simulink model "flightControlSystem"  (R2021a)
settings: Solver=ode3  StartTime=0  StopTime=TFinal  FixedStep=Ts  RelTol=1e-3  EnableMultiTasking=on
undefined symbols (not defined in the file): BINARIZATION_THRESHOLD, CHANGE_DERIVATIVE_ERROR_THRESHOLD_CURVE, CHANGE_DERIVATIVE_ERROR_THRESHOLD_STRAIGHT, codertarget, COG_X, COG_Y, Controller, DELAY_LANDING, DERIVATIVE_GAIN, DILATE_KERNEL, DiscIntNeverNeededParam, Discrete, DISK_KERNEL, Estimator, FLAG_WAIT_FOR_HOVERING, FOV_CURVE, FOV_STRAIGHT, FRAME_SIZE_HEIGHT, FRAME_SIZE_WIDTH, g, G_B_GAIN, GAIN_LANDING, GAIN_TRACK, init, MAX_RADIUS_CROWN_CURVE, MAX_RADIUS_CROWN_STRAIGHT, MIN_RADIUS_CROWN_CURVE, MIN_RADIUS_CROWN_STRAIGHT, Sensors, strel, Time, TIME_HOLD, Ts, var_acc_angle_N, var_bias_gyr_N, var_gyro_p_N, Vehicle, Z_HIGH, Z_LOW
libraries: simulink x39, ctrlSharedLib x4, sharedtransform x3, visionmorphops x2, parrotlib x1
(part 2 of 3)

== system flightControlSystem/Control System/State Estimator/XY Position Estimator ==
  opticalFlow_datin : Inport
  controlModePosVSOrient_flagin : Inport  Port=2
  sensorIMU_datin : Inport  Port=3
  Z_estimin : Inport  Port=4
  dz_estimin : Inport  Port=5
  orient_estimin : Inport  Port=6
  Angular velocity : Inport  Port=7
  EstimatorVelocity : Subsystem
  EstimatorXYPosition : Subsystem
  XY_estimout : Outport  VectorParamsAs1DForOutWhenUnconnected=off
  dxy_estimout : Outport  Port=2  VectorParamsAs1DForOutWhenUnconnected=off
  wires:
  EstimatorXYPosition/1(XY_estimout) -> XY_estimout/1
  dz_estimin/1 -> EstimatorXYPosition/4(dz_estimin)
  controlModePosVSOrient_flagin/1 -> EstimatorXYPosition/3(controlModePosVSOrient_flagin)
  Z_estimin/1 -> EstimatorVelocity/2(Z_estimin)
  sensorIMU_datin/1 -> EstimatorVelocity/3(sensorIMU_datin)
  opticalFlow_datin/1 -> EstimatorVelocity/1(opticalFlow_datin)
  EstimatorVelocity/1(dxy_estimout) -> dxy_estimout/1, EstimatorXYPosition/1(dxy_estimin)
  orient_estimin/1 -> EstimatorXYPosition/2(orient_estimin), EstimatorVelocity/4(orient_estimin)
  Angular velocity/1 -> EstimatorVelocity/5(angular velocity)

== system flightControlSystem/Control System/Path Planning/Non linear Path Planner/X_PLANNER ==
  x_estimated : Inport
  error_x : Inport  Port=2
  flag_end_marker : Inport  Port=3
  flag_end_marker_to_controller : Inport  Port=4
  flag_track : Inport  Port=5
  flag_hover : Inport  Port=6
  change_threshold : Inport  Port=7
  Cast To Double1 : DataTypeConversion  OutDataTypeStr=double
  Chart1 : Stateflow chart  TreatAsAtomicUnit=on
  "x_derivative_contribute " : Subsystem
  x_linear_contribute : Stateflow chart  TreatAsAtomicUnit=on
  x_planned : Outport  VectorParamsAs1DForOutWhenUnconnected=off
  wires:
  "x_derivative_contribute "/1(derivative_x_part) -> Chart1/1(dev_part)
  x_estimated/1 -> Cast To Double1/1
  flag_end_marker_to_controller/1 -> Chart1/3(flag_end_marker_to_controller)
  error_x/1 -> "x_derivative_contribute "/1(error_x), x_linear_contribute/1(error)
  Cast To Double1/1 -> Chart1/4(x_estimated)
  flag_track/1 -> Chart1/5(flag_track), x_linear_contribute/3(flag_track)
  x_linear_contribute/1(linear_part) -> Chart1/2(lin_part)
  flag_end_marker/1 -> Chart1/6(flag_end_marker), x_linear_contribute/2(flag_end_marker)
  Chart1/1(x_planned) -> x_planned/1
  flag_hover/1 -> Chart1/7(flag_hover)
  change_threshold/1 -> "x_derivative_contribute "/2(change_threshold)

== system flightControlSystem/Control System/Path Planning/Non linear Path Planner/Y_PLANNER ==
  flag_track : Inport
  flag_end_marker_to_controller : Inport  Port=2
  flag_end_marker : Inport  Port=3
  error_y : Inport  Port=4
  y_estimated : Inport  Port=5
  flag_hover : Inport  Port=6
  change_threshold : Inport  Port=7
  Cast To Double1 : DataTypeConversion  OutDataTypeStr=double
  Chart1 : Stateflow chart  TreatAsAtomicUnit=on
  "y_derivative_contribute " : Subsystem
  y_linear_contribute : Stateflow chart  TreatAsAtomicUnit=on
  y_planned : Outport  VectorParamsAs1DForOutWhenUnconnected=off
  wires:
  error_y/1 -> y_linear_contribute/1(error), "y_derivative_contribute "/2(error_y)
  "y_derivative_contribute "/1(derivative_y_part) -> Chart1/1(dev_part)
  y_estimated/1 -> Cast To Double1/1
  flag_end_marker/1 -> Chart1/5(flag_end_marker), y_linear_contribute/2(flag_end_marker)
  flag_track/1 -> Chart1/4(flag_track), y_linear_contribute/3(flag_track)
  y_linear_contribute/1(linear_part) -> Chart1/2(lin_part)
  Cast To Double1/1 -> Chart1/6(y_estimated)
  flag_end_marker_to_controller/1 -> Chart1/3(flag_end_marker_to_controller)
  Chart1/1(y_planned) -> y_planned/1
  flag_hover/1 -> Chart1/7(flag_hover)
  change_threshold/1 -> "y_derivative_contribute "/1(change_threshold)

== system flightControlSystem/Control System/Path Planning/Non linear Path Planner/Z PLANNER ==
  error_x : Inport
  flag_end_marker : Inport  Port=2
  error_y : Inport  Port=3
  flag_hover : Inport  Port=4
  Chart : Stateflow chart  TreatAsAtomicUnit=on
  Delay1 : Delay  DelayLength=DELAY_LANDING
  Display : Display
  MATLAB Function : MATLAB Function  TreatAsAtomicUnit=on
  z_planned : Outport  VectorParamsAs1DForOutWhenUnconnected=off
  flag_end_marker_to_controller : Outport  Port=2  VectorParamsAs1DForOutWhenUnconnected=off
  wires:
  error_y/1 -> MATLAB Function/2(error_y)
  error_x/1 -> MATLAB Function/1(error_x)
  flag_end_marker/1 -> Chart/2(flag_end_marker), MATLAB Function/3(flag_end_marker)
  MATLAB Function/2(norm_error) -> Delay1/1
  Delay1/1 -> MATLAB Function/4(norm_error_prev)
  MATLAB Function/1(norm_error_tot) -> Display/1, Chart/1(norm_error)
  Chart/1(z_planned) -> z_planned/1
  Chart/2(flag_end_marker_to_controller) -> flag_end_marker_to_controller/1
  flag_hover/1 -> Chart/3(flag_hover)

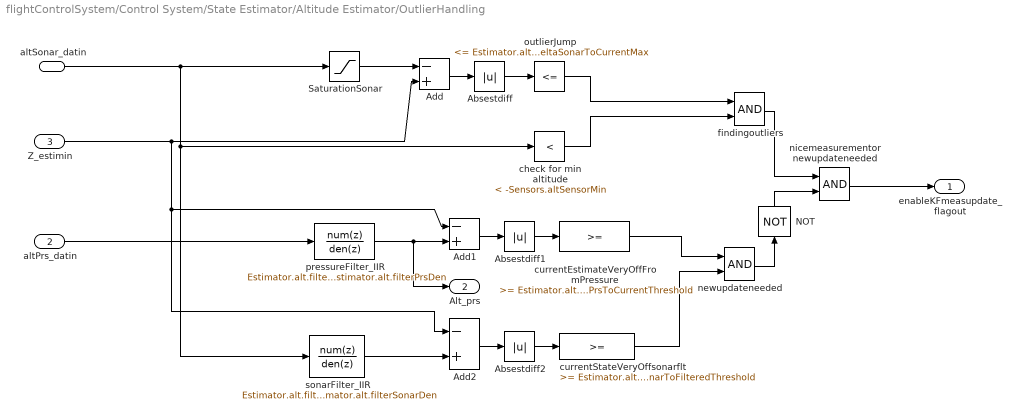
== system flightControlSystem/Control System/State Estimator/Altitude Estimator/OutlierHandling ==
  altSonar_datin : Inport
  altPrs_datin : Inport  Port=2
  Z_estimin : Inport  Port=3
  Absestdiff : Abs
  Absestdiff1 : Abs
  Absestdiff2 : Abs
  Add : Sum  Inputs=-+
  Add1 : Sum  Inputs=-+
  Add2 : Sum  Inputs=-+
  NOT : Logic  Operator=NOT  IconShape=distinctive  AllPortsSameDT=off  OutDataTypeStr=boolean
  SaturationSonar : Saturate  UpperLimit=-Sensors.altSensorMin  LowerLimit=-inf
  check for min altitude : simulink/Logic and Bit Operations/Compare To Constant  relop=<  const=-Sensors.altSensorMin  OutDataTypeStr=boolean
  currentEstimateVeryOffFromPressure : simulink/Logic and Bit Operations/Compare To Constant  relop=>=  const=Estimator.alt.deltaPrsToCurrentThreshold  OutDataTypeStr=boolean
  currentStateVeryOffsonarflt : simulink/Logic and Bit Operations/Compare To Constant  relop=>=  const=Estimator.alt.deltaSonarToFilteredThreshold  OutDataTypeStr=boolean
  findingoutliers : Logic  AllPortsSameDT=off  OutDataTypeStr=boolean
  newupdateneeded : Logic  AllPortsSameDT=off  OutDataTypeStr=boolean
  nicemeasurementor newupdateneeded : Logic  AllPortsSameDT=off  OutDataTypeStr=boolean
  outlierJump : simulink/Logic and Bit Operations/Compare To Constant  relop=<=  const=Estimator.alt.deltaSonarToCurrentMax  OutDataTypeStr=boolean
  pressureFilter_IIR : DiscreteFilter  Numerator=Estimator.alt.filterPrsNum  Denominator=Estimator.alt.filterPrsDen
  sonarFilter_IIR : DiscreteFilter  Numerator=Estimator.alt.filterSonarNum  Denominator=Estimator.alt.filterSonarDen
  enableKFmeasupdate_flagout : Outport  VectorParamsAs1DForOutWhenUnconnected=off
  Alt_prs : Outport  Port=2  VectorParamsAs1DForOutWhenUnconnected=off
  wires:
  Add1/1 -> Absestdiff1/1
  nicemeasurementor newupdateneeded/1 -> enableKFmeasupdate_flagout/1
  findingoutliers/1 -> nicemeasurementor newupdateneeded/1
  check for min altitude/1 -> findingoutliers/2
  outlierJump/1 -> findingoutliers/1
  SaturationSonar/1 -> Add/1
  Absestdiff/1 -> outlierJump/1
  Add/1 -> Absestdiff/1
  newupdateneeded/1 -> NOT/1
  Absestdiff2/1 -> currentStateVeryOffsonarflt/1
  altSonar_datin/1 -> SaturationSonar/1, sonarFilter_IIR/1, check for min altitude/1
  currentEstimateVeryOffFromPressure/1 -> newupdateneeded/1
  Z_estimin/1 -> Add1/1, Add2/1, Add/2
  Add2/1 -> Absestdiff2/1
  currentStateVeryOffsonarflt/1 -> newupdateneeded/2
  pressureFilter_IIR/1 -> Alt_prs/1, Add1/2
  altPrs_datin/1 -> pressureFilter_IIR/1
  sonarFilter_IIR/1 -> Add2/2
  Absestdiff1/1 -> currentEstimateVeryOffFromPressure/1
  NOT/1 -> nicemeasurementor newupdateneeded/2

== system flightControlSystem/Control System/State Estimator/Attitude Estimator/Pitch_Kalman ==
  note: Gyroscope's bias is susceptible to factors like "temperature" and "Gyro bias stability" and it
      | can vary during the flight. It is therefore estimated using this Kalman filter making use of Accelerometer data
  note: Linear Kalman filter is used for the Pitch and Roll estimation.
      | The states are the corresponding Euler angle and Angular rate bias respectively
  axyz : Inport
  pitch_rate : Inport  Port=2
  enable_update : Inport  Port=3
  Demux : Demux  Outputs=2
  Gain2 : Gain  Gain=1/g
  Kalman Filter : ctrlSharedLib/Kalman Filter  TimeDomain=Discrete-Time  UseCurrentEstimator=on  ModelSource=Individual A, B, C, D matrices  ModelSourceVariable=ss(0.95,1,1,0,1)  A=[1 -Ts;0 1]  B=[Ts;0]  C=[1 0]  D=0  NumberOfStates=1  NumberOfInputs=1  NumberOfOutputs=1  InitialEstimateSource=Dialog  X0=0  P0=10  UseK=off  UseGH=off  NumberOfProcessNoiseInputs=1  G=1  TimeInvariantG=on  H=0  TimeInvariantH=on  Q=[var_gyro_p_N,0;0,var_bias_gyr_N]  TimeInvariantQ=on  R=var_acc_angle_N  TimeInvariantR=on  N=0  TimeInvariantN=on  AddInputPort=on  AddEnablePort=on  OutputEstimatedY=off  OutputP=off  Ts=Ts
  Selector1 : Selector  InputPortWidth=3  IndexOptions=Index vector (dialog)  Indices=[1]  OutputSizes=1
  Trigonometric Function1 : Trigonometry  Operator=asin
  single : DataTypeConversion  OutDataTypeStr=single
  single1 : DataTypeConversion  OutDataTypeStr=single
  pitch : Outport
  gyro_y_bias : Outport  Port=2
  wires:
  Kalman Filter/1 -> Demux/1
  Demux/1 -> single1/1
  Gain2/1 -> Trigonometric Function1/1
  Trigonometric Function1/1 -> Kalman Filter/2
  Selector1/1 -> Gain2/1
  axyz/1 -> Selector1/1
  pitch_rate/1 -> Kalman Filter/1
  enable_update/1 -> Kalman Filter/3
  Demux/2 -> single/1
  single/1 -> gyro_y_bias/1
  single1/1 -> pitch/1

== system flightControlSystem/Control System/State Estimator/Attitude Estimator/Roll_Kalman ==
  note: Linear Kalman filter is used for the Pitch and Roll estimation.
      | The states are the corresponding Euler angle and Angular rate bias respectively
  note: Gyroscope's bias is susceptible to factors like "temperature" and "Gyro bias stability" and it
      | can vary during the flight. It is therefore estimated using the Kalman filter making use of accelerometer data
  axyz : Inport
  roll_rate : Inport  Port=2
  enable_update : Inport  Port=3
  Data Type Conversion : DataTypeConversion
  Data Type Conversion1 : DataTypeConversion
  Demux : Demux  Outputs=3
  Demux1 : Demux  Outputs=2
  Divide : Product  Inputs=*/
  Kalman Filter : ctrlSharedLib/Kalman Filter  TimeDomain=Discrete-Time  UseCurrentEstimator=on  ModelSource=Individual A, B, C, D matrices  ModelSourceVariable=ss(0.95,1,1,0,1)  A=[1 -Ts;0 1]  B=[Ts;0]  C=[1 0]  D=0  NumberOfStates=1  NumberOfInputs=1  NumberOfOutputs=1  InitialEstimateSource=Dialog  X0=0  P0=10  UseK=off  UseGH=off  NumberOfProcessNoiseInputs=1  G=1  TimeInvariantG=on  H=0  TimeInvariantH=on  Q=[var_gyro_p_N,0;0,var_bias_gyr_N]  TimeInvariantQ=on  R=var_acc_angle_N  TimeInvariantR=on  N=0  TimeInvariantN=on  AddInputPort=on  AddEnablePort=on  OutputEstimatedY=off  OutputP=off  Ts=Ts
  Terminator : Terminator
  Trigonometric Function : Trigonometry  Operator=atan
  roll : Outport
  gyro_x_bias : Outport  Port=2
  wires:
  Demux1/1 -> Data Type Conversion1/1
  Kalman Filter/1 -> Demux1/1
  roll_rate/1 -> Kalman Filter/1
  Divide/1 -> Trigonometric Function/1
  Demux/2 -> Divide/1
  axyz/1 -> Demux/1
  Demux/3 -> Divide/2
  Trigonometric Function/1 -> Kalman Filter/2
  enable_update/1 -> Kalman Filter/3
  Demux1/2 -> Data Type Conversion/1
  Data Type Conversion/1 -> gyro_x_bias/1
  Data Type Conversion1/1 -> roll/1
  Demux/1 -> Terminator/1

== system flightControlSystem/Control System/State Estimator/Attitude Estimator/Yaw_integrator ==
  note: Yaw angle is not constrained between -180 to 180 degrees
  note: Currently yaw angle is obtained solely by integrating the gyroscope output.
      | This yaw estimate can drift with time.
  yaw_rate : Inport
  Constant : Constant  Value=0  OutDataTypeStr=single
  Discrete-Time Integrator : DiscreteIntegrator  SampleTime=-1  ICPrevOutput=DiscIntNeverNeededParam  ICPrevScaledInput=DiscIntNeverNeededParam
  yaw : Outport
  gyro_z_bias : Outport  Port=2
  wires:
  yaw_rate/1 -> Discrete-Time Integrator/1
  Discrete-Time Integrator/1 -> yaw/1
  Constant/1 -> gyro_z_bias/1

== system flightControlSystem/Control System/State Estimator/Attitude Estimator/norm(accelerometer) ==
  In1 : Inport
  Constant : Constant  Value=2  OutDataTypeStr=single
  Data Type Conversion2 : DataTypeConversion  OutDataTypeStr=single
  Math Function : Math  Operator=pow  SignedPower=on  SaturateOnIntegerOverflow=on
  Sqrt : Sqrt  SaturateOnIntegerOverflow=on
  Sum of Elements : Sum  Inputs=+
  Out1 : Outport
  wires:
  Sum of Elements/1 -> Sqrt/1
  Math Function/1 -> Sum of Elements/1
  Data Type Conversion2/1 -> Math Function/1
  In1/1 -> Data Type Conversion2/1
  Constant/1 -> Math Function/2
  Sqrt/1 -> Out1/1

== system flightControlSystem/Control System/State Estimator/SensorPreprocessing/Temperature Compensation ==
  note: Gyroscope's bias is affected by temperature.This won't be a problem for Pitch and Roll angle estimation as the actual gyroscope bias in the Pitch and Roll axis are estimated during the flight. However the yaw orientation is obtained by integrating the gyroscope output and it may drift with time. Even the preflight calibration which is done cannot compensate for this problem as the gyro bis varies during the flight.
  Gyro Temperature : Inport
  uncompensated_gyro_z_rate : Inport  Port=2
  Compare To Constant : simulink/Logic and Bit Operations/Compare To Constant  relop===  const=1  OutDataTypeStr=boolean
  Constant : Constant  Value=0
  Counter Free-Running : simulink/Sources/Counter Free-Running  NumBits=32  tsamp=0.005
  Data Type Conversion1 : DataTypeConversion
  Disable temperature compensation : ManualSwitch
  Gain : Gain  Gain=0.00228
  Subtract : Sum  Inputs=+-
  Subtract1 : Sum  Inputs=+-
  Triggered Subsystem : Subsystem  TreatAsAtomicUnit=on
  r : Outport
  wires:
  Gain/1 -> Disable temperature compensation/1
  Disable temperature compensation/1 -> Data Type Conversion1/1
  Gyro Temperature/1 -> Subtract/1, Triggered Subsystem/1(In1)
  Triggered Subsystem/1(Out1) -> Subtract/2  "Initial temperature"
  Compare To Constant/1 -> Triggered Subsystem/Trigger
  Constant/1 -> Disable temperature compensation/2
  Subtract/1 -> Gain/1
  Data Type Conversion1/1 -> Subtract1/2
  Counter Free-Running/1 -> Compare To Constant/1
  uncompensated_gyro_z_rate/1 -> Subtract1/1
  Subtract1/1 -> r/1  "r"

== system flightControlSystem/Control System/State Estimator/SensorPreprocessing/sensordata_group ==
  HAL_acc_SI : Inport  OutDataTypeStr=Bus: HAL_acc_SI_t
  HAL_gyro_SI : Inport  Port=2  OutDataTypeStr=Bus: HAL_gyro_SI_t
  HAL_ultrasound_SI : Inport  Port=3  OutDataTypeStr=Bus: HAL_ultrasound_SI_t
  HAL_pressure_SI : Inport  Port=4  OutDataTypeStr=Bus: HAL_pressure_SI_t
  HAL_vbat_SI : Inport  Port=5  OutDataTypeStr=Bus: HAL_vbat_SI_t
  Bus Selector1 : BusSelector  OutputSignals=vbat_V,vbat_percentage
  Bus Selector3 : BusSelector  OutputSignals=x,y,z
  Bus Selector4 : BusSelector  OutputSignals=x,y,z,temperature
  Bus Selector5 : BusSelector  OutputSignals=altitude
  Bus Selector6 : BusSelector  OutputSignals=pressure
  Out Bus Element : Outport  VectorParamsAs1DForOutWhenUnconnected=off  PortName=sensordata_datin  Element=ddx
  Out Bus Element1 : Outport  VectorParamsAs1DForOutWhenUnconnected=off  PortName=sensordata_datin  Element=ddy
  Out Bus Element2 : Outport  VectorParamsAs1DForOutWhenUnconnected=off  PortName=sensordata_datin  Element=ddz
  Out Bus Element3 : Outport  VectorParamsAs1DForOutWhenUnconnected=off  PortName=sensordata_datin  Element=p
  Out Bus Element4 : Outport  VectorParamsAs1DForOutWhenUnconnected=off  PortName=sensordata_datin  Element=q
  Out Bus Element5 : Outport  VectorParamsAs1DForOutWhenUnconnected=off  PortName=sensordata_datin  Element=r
  Out Bus Element6 : Outport  VectorParamsAs1DForOutWhenUnconnected=off  PortName=sensordata_datin  Element=altitude_sonar
  Out Bus Element7 : Outport  VectorParamsAs1DForOutWhenUnconnected=off  PortName=sensordata_datin  Element=prs
  Out Bus Element8 : Outport  VectorParamsAs1DForOutWhenUnconnected=off  PortName=sensordata_datin  Element=vbat_V
  Out Bus Element9 : Outport  VectorParamsAs1DForOutWhenUnconnected=off  PortName=sensordata_datin  Element=vbat_percentage
  Out1 : Outport  Port=2
  wires:
  HAL_gyro_SI/1 -> Bus Selector4/1
  HAL_acc_SI/1 -> Bus Selector3/1
  HAL_pressure_SI/1 -> Bus Selector6/1
  HAL_ultrasound_SI/1 -> Bus Selector5/1
  Bus Selector4/1 -> Out Bus Element3/1  "<x>"
  Bus Selector3/3 -> Out Bus Element2/1  "<z>"
  Bus Selector4/3 -> Out Bus Element5/1  "<z>"
  Bus Selector5/1 -> Out Bus Element6/1  "<altitude>"
  Bus Selector6/1 -> Out Bus Element7/1  "<pressure>"
  Bus Selector4/2 -> Out Bus Element4/1  "<y>"
  Bus Selector3/1 -> Out Bus Element/1  "<x>"
  Bus Selector3/2 -> Out Bus Element1/1  "<y>"
  Bus Selector1/1 -> Out Bus Element8/1  "<vbat_V>"
  HAL_vbat_SI/1 -> Bus Selector1/1
  Bus Selector1/2 -> Out Bus Element9/1  "<vbat_percentage>"
  Bus Selector4/4 -> Out1/1  "<temperature>"

== system flightControlSystem/Control System/State Estimator/XY Position Estimator/EstimatorVelocity ==
  opticalFlow_datin : Inport
  Z_estimin : Inport  Port=2  SampleTime=Ts
  sensorIMU_datin : Inport  Port=3
  orient_estimin : Inport  Port=4
  angular velocity : Inport  Port=5
  AccelerationHandling : Subsystem
  Angular velocity compensation for optical flow : Subsystem
  DataHandling : Subsystem
  Delay : Delay  DelayLength=1  InitialCondition=0
  KalmanFilter_dxdy : ctrlSharedLib/Kalman Filter  TimeDomain=Discrete-Time  UseCurrentEstimator=on  ModelSource=Individual A, B, C, D matrices  ModelSourceVariable=ss(0.95,1,1,0,1)  A=Estimator.pos.kfVelo.A  B=Estimator.pos.kfVelo.B  C=Estimator.pos.kfVelo.C  D=Estimator.pos.kfVelo.D  NumberOfStates=1  NumberOfInputs=1  NumberOfOutputs=1  InitialEstimateSource=Dialog  X0=0  P0=10  UseK=off  UseGH=off  NumberOfProcessNoiseInputs=1  G=Estimator.pos.kfVelo.G  TimeInvariantG=on  H=Estimator.pos.kfVelo.H  TimeInvariantH=on  Q=Estimator.pos.kfVelo.Q  TimeInvariantQ=on  R=Estimator.pos.kfVelo.R  TimeInvariantR=on  N=Estimator.pos.kfVelo.N  TimeInvariantN=on  AddInputPort=on  AddEnablePort=on  OutputEstimatedY=off  OutputP=off  Ts=-1
  Selector1 : Selector  InputPortWidth=4  IndexOptions=Index vector (dialog)  Indices=[1 2]  OutputSizes=1
  Z_estimin1 : InportShadow  Port=2  SampleTime=Ts
  angular velocity compensation : Sum
  xy velocity w/o angular velocity compensation : Subsystem
  dxy_estimout : Outport  VectorParamsAs1DForOutWhenUnconnected=off
  wires:
  Z_estimin/1 -> DataHandling/1(Z_estimin), AccelerationHandling/4(Z_estimin)
  KalmanFilter_dxdy/1 -> Selector1/1
  sensorIMU_datin/1 -> AccelerationHandling/2(sensorIMU_datin), DataHandling/3(sensorIMU_datin)
  orient_estimin/1 -> AccelerationHandling/3(orient_estimin), DataHandling/2(orient_estimin)
  Z_estimin1/1 -> xy velocity w/o angular velocity compensation/2(z_estimate), Angular velocity compensation for optical flow/1(z_estimate)
  AccelerationHandling/1(acceleration_world) -> KalmanFilter_dxdy/1
  angular velocity compensation/1 -> KalmanFilter_dxdy/2
  Delay/1 -> DataHandling/5(dxyOF_datin)
  Selector1/1 -> dxy_estimout/1, Delay/1
  angular velocity/1 -> Angular velocity compensation for optical flow/2(Angular velocity w/o bias)
  Angular velocity compensation for optical flow/1(angular velocity correction) -> angular velocity compensation/2
  xy velocity w/o angular velocity compensation/1(optical_flow_dx_dy) -> DataHandling/4(dxy_estimin), AccelerationHandling/1(dxy_estimin), angular velocity compensation/1
  opticalFlow_datin/1 -> xy velocity w/o angular velocity compensation/1(optical_flow)
  DataHandling/1(enable_flag) -> KalmanFilter_dxdy/3

== system flightControlSystem/Control System/State Estimator/XY Position Estimator/EstimatorXYPosition ==
  note: Switching from orientationControl to Position
      | control reset the current world position estimate
      | (happens when using no markers)
  dxy_estimin : Inport
  orient_estimin : Inport  Port=2  SampleTime=Ts
  controlModePosVSOrient_flagin : Inport  Port=3
  dz_estimin : Inport  Port=4
  Math Function : Math  Operator=transpose  SignedPower=on  SaturateOnIntegerOverflow=on
  Mux2 : Mux  Inputs=2
  Product : Product  Multiplication=Matrix(*)
  Rotation Angles to Direction Cosine Matrix : sharedtransform/Rotation Angles to Direction Cosine Matrix  rotationOrder=ZYX  aMode=aMode
      settings: SourceProductBaseCode=AE,PW,DR,MT,UV,VE
  SelectdXY : Selector  InputPortWidth=3  IndexOptions=Index vector (dialog)  Indices=[1 2]  OutputSizes=1
  SimplyIntegrateVelocity : DiscreteIntegrator  ExternalReset=rising  SampleTime=Ts  ICPrevOutput=DiscIntNeverNeededParam  ICPrevScaledInput=DiscIntNeverNeededParam
  XY_estimout : Outport  VectorParamsAs1DForOutWhenUnconnected=off
  wires:
  controlModePosVSOrient_flagin/1 -> SimplyIntegrateVelocity/2
  Product/1 -> SelectdXY/1
  Mux2/1 -> Product/2
  dz_estimin/1 -> Mux2/2
  SimplyIntegrateVelocity/1 -> XY_estimout/1
  dxy_estimin/1 -> Mux2/1
  orient_estimin/1 -> Rotation Angles to Direction Cosine Matrix/1
  Rotation Angles to Direction Cosine Matrix/1 -> Math Function/1
  SelectdXY/1 -> SimplyIntegrateVelocity/1
  Math Function/1 -> Product/1

== system flightControlSystem/Control System/Path Planning/Non linear Path Planner/X_PLANNER/x_derivative_contribute  ==
  error_x : Inport
  change_threshold : Inport  Port=2
  Delay : Delay  DelayLength=1  InitialCondition=0
  Delay5 : Delay  DelayLength=1
  Delay6 : Delay  DelayLength=1  InitialCondition=0
  Discrete Derivative : simulink/Discrete/Discrete Derivative  gainval=Ts  ICPrevScaledInput=0.0  OutMin=[]  OutMax=[]  OutDataType=fixdt(1, 16)  OutScaling=2^-10  DoSatur=off
  MATLAB Function : MATLAB Function  TreatAsAtomicUnit=on
  derivative error : MATLAB Function  TreatAsAtomicUnit=on
  derivative_x_part : Outport  VectorParamsAs1DForOutWhenUnconnected=off
  wires:
  error_x/1 -> Discrete Derivative/1
  derivative error/3(flag_count) -> Delay5/1
  derivative error/2(count) -> Delay/1
  Delay/1 -> derivative error/4(count_prev)
  Discrete Derivative/1 -> derivative error/2(derivative_error), MATLAB Function/1(derivative_error)  "derivative_error"
  Delay5/1 -> derivative error/5(flag_count_prev)
  MATLAB Function/1(flag_change_error) -> derivative error/3(flag_change_error)  "flag_change_error"
  derivative error/1(dev_contribute) -> Delay6/1, derivative_x_part/1
  Delay6/1 -> derivative error/1(dev_contribute_prev)
  change_threshold/1 -> MATLAB Function/2(CHANGE_DERIVATIVE_ERROR_THRESHOLD)

== system flightControlSystem/Control System/Path Planning/Non linear Path Planner/Y_PLANNER/y_derivative_contribute  ==
  change_threshold : Inport
  error_y : Inport  Port=2
  Delay : Delay  DelayLength=1  InitialCondition=0
  Delay5 : Delay  DelayLength=1
  Delay6 : Delay  DelayLength=1  InitialCondition=0
  Discrete Derivative : simulink/Discrete/Discrete Derivative  gainval=Ts  ICPrevScaledInput=0.0  OutMin=[]  OutMax=[]  OutDataType=fixdt(1, 16)  OutScaling=2^-10  DoSatur=off
  MATLAB Function : MATLAB Function  TreatAsAtomicUnit=on
  derivative error : MATLAB Function  TreatAsAtomicUnit=on
  derivative_y_part : Outport  VectorParamsAs1DForOutWhenUnconnected=off
  wires:
  error_y/1 -> Discrete Derivative/1
  derivative error/3(flag_count) -> Delay5/1
  derivative error/2(count) -> Delay/1
  Delay/1 -> derivative error/4(count_prev)
  Delay5/1 -> derivative error/5(flag_count_prev)
  MATLAB Function/1(flag_change_error) -> derivative error/3(flag_change_error)
  derivative error/1(dev_contribute) -> Delay6/1, derivative_y_part/1
  Delay6/1 -> derivative error/1(dev_contribute_prev)
  change_threshold/1 -> MATLAB Function/2(CHANGE_DERIVATIVE_ERROR_THRESHOLD)
  Discrete Derivative/1 -> derivative error/2(derivative_error), MATLAB Function/1(derivative_error)

== system flightControlSystem/Control System/State Estimator/SensorPreprocessing/Temperature Compensation/Triggered Subsystem ==
  In1 : Inport
  Trigger : TriggerPort  TriggerType=either  VariantControl=Variant
  Out1 : Outport
  wires:
  In1/1 -> Out1/1

== system flightControlSystem/Control System/State Estimator/XY Position Estimator/EstimatorVelocity/AccelerationHandling ==
  dxy_estimin : Inport
  sensorIMU_datin : Inport  Port=2
  orient_estimin : Inport  Port=3
  Z_estimin : Inport  Port=4
  Add : Sum  Inputs=-+
  Bus Selector1 : BusSelector  OutputSignals=ddx,ddy,ddz
  Deactivate Acceleration If OF is not used due to low altitude : simulink/Logic and Bit Operations/Compare To Constant  relop=<=  const=Estimator.pos.opticalFlowZMax  OutDataTypeStr=boolean
  Logical Operator : Logic  Operator=OR  AllPortsSameDT=off  OutDataTypeStr=boolean
  Mux6 : Mux  Inputs=3
  Product : Product  Inputs=3
  Product1 : Product  Multiplication=Matrix(*)
  Rotation Angles to Direction Cosine Matrix : sharedtransform/Rotation Angles to Direction Cosine Matrix  rotationOrder=ZYX  aMode=aMode
      settings: SourceProductBaseCode=AE,PW,DR,MT,UV,VE
  SelectPlanarddxy : Selector  InputPortWidth=3  IndexOptions=Index vector (dialog)  Indices=[1 2]  OutputSizes=1
  Selector : Selector  InputPortWidth=2  IndexOptions=Index vector (dialog)  Indices=1  OutputSizes=1
  Selector1 : Selector  InputPortWidth=2  IndexOptions=Index vector (dialog)  Indices=2  OutputSizes=1
  do not use acc if optical flow never available (Note OF@60Hz but ZOH to 200!) : simulink/Logic and Bit Operations/Compare To Constant  relop=~=  const=0  OutDataTypeStr=boolean
  do not use acc if optical flow never available (Note OF@60Hz but ZOH to 200!)1 : simulink/Logic and Bit Operations/Compare To Constant  relop=~=  const=0  OutDataTypeStr=boolean
  gainaccinput1 : Gain  OutDataTypeStr=single
  gravity : Constant  Value=[0 0 -g]
  acceleration_world : Outport  OutDataTypeStr=single  VectorParamsAs1DForOutWhenUnconnected=off
  wires:
  do not use acc if optical flow never available (Note OF@60Hz but ZOH to 200!)1/1 -> Logical Operator/2
  do not use acc if optical flow never available (Note OF@60Hz but ZOH to 200!)/1 -> Logical Operator/1
  Logical Operator/1 -> Product/1
  Selector1/1 -> do not use acc if optical flow never available (Note OF@60Hz but ZOH to 200!)1/1
  Selector/1 -> do not use acc if optical flow never available (Note OF@60Hz but ZOH to 200!)/1
  dxy_estimin/1 -> Selector1/1, Selector/1
  Product/1 -> acceleration_world/1
  Deactivate Acceleration If OF is not used due to low altitude/1 -> Product/3
  Z_estimin/1 -> Deactivate Acceleration If OF is not used due to low altitude/1
  Add/1 -> SelectPlanarddxy/1
  Product1/1 -> Add/1
  gravity/1 -> Product1/2
  SelectPlanarddxy/1 -> gainaccinput1/1
  Bus Selector1/3 -> Mux6/3  "<ddz>"
  Bus Selector1/1 -> Mux6/1  "<ddx>"
  sensorIMU_datin/1 -> Bus Selector1/1
  Mux6/1 -> Add/2
  Bus Selector1/2 -> Mux6/2  "<ddy>"
  orient_estimin/1 -> Rotation Angles to Direction Cosine Matrix/1
  Rotation Angles to Direction Cosine Matrix/1 -> Product1/1
  gainaccinput1/1 -> Product/2

== system flightControlSystem/Control System/State Estimator/XY Position Estimator/EstimatorVelocity/Angular velocity compensation for optical flow ==
  note: Optical flow readings are affected by both linear and angular velocity of the drone. We need to subtract the effect of angular velocity before using the flow data
  z_estimate : Inport
  Angular velocity w/o bias : Inport  Port=2
  Abs : Abs
  Data Type Conversion : DataTypeConversion
  Demux : Demux  Outputs=2
  Gain1 : Gain  Gain=-1
  Mux : Mux  Inputs=2
  Selector : Selector  InputPortWidth=3  IndexOptions=Index vector (dialog)  Indices=[1 2]  OutputSizes=1
  prod : Product  Inputs=**
  angular velocity correction : Outport
  wires:
  Gain1/1 -> Mux/1
  Mux/1 -> Data Type Conversion/1
  Demux/2 -> Gain1/1
  Data Type Conversion/1 -> angular velocity correction/1
  prod/1 -> Demux/1
  z_estimate/1 -> Abs/1
  Demux/1 -> Mux/2
  Selector/1 -> prod/2
  Abs/1 -> prod/1
  Angular velocity w/o bias/1 -> Selector/1

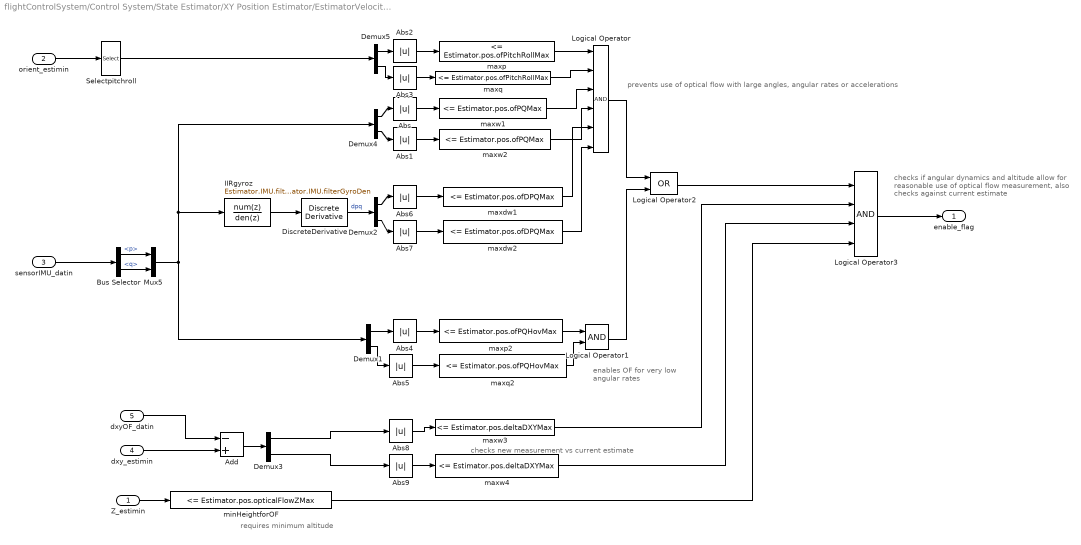
== system flightControlSystem/Control System/State Estimator/XY Position Estimator/EstimatorVelocity/DataHandling ==
  note: prevents use of optical flow with large angles, angular rates or accelerations
  note: enables OF for very
      | low angular rates
  note: checks if angular dynamics and altitude allow for
      | reasonable use of optical flow measurement,
      | also checks against current estimate
  note: checks new measurement vs current estimate
  note: requires minimum altitude
  Z_estimin : Inport
  orient_estimin : Inport  Port=2
  sensorIMU_datin : Inport  Port=3
  dxy_estimin : Inport  Port=4
  dxyOF_datin : Inport  Port=5
  Abs{,1..9} (10 alike) : Abs
  Add : Sum  Inputs=-+
  Bus Selector : BusSelector  OutputSignals=p,q
  Demux{1..5} (5 alike) : Demux  Outputs=2
  DiscreteDerivative : simulink/Discrete/Discrete Derivative  gainval=1.0  ICPrevScaledInput=0.0  OutMin=[]  OutMax=[]  OutDataType=fixdt(1, 16)  OutScaling=2^-10  DoSatur=off
  IIRgyroz : DiscreteFilter  Numerator=Estimator.IMU.filterGyroNum  Denominator=Estimator.IMU.filterGyroDen
  Logical Operator : Logic  Inputs=6  AllPortsSameDT=off  OutDataTypeStr=boolean
  Logical Operator1 : Logic  AllPortsSameDT=off  OutDataTypeStr=boolean
  Logical Operator2 : Logic  Operator=OR  AllPortsSameDT=off  OutDataTypeStr=boolean
  Logical Operator3 : Logic  Inputs=4  AllPortsSameDT=off  OutDataTypeStr=boolean
  Mux5 : Mux  Inputs=2
  Selectpitchroll : Selector  InputPortWidth=3  IndexOptions=Index vector (dialog)  Indices=[2 3]  OutputSizes=1
  maxdw1 : simulink/Logic and Bit Operations/Compare To Constant  relop=<=  const=Estimator.pos.ofDPQMax  OutDataTypeStr=boolean
  maxdw2 : simulink/Logic and Bit Operations/Compare To Constant  relop=<=  const=Estimator.pos.ofDPQMax  OutDataTypeStr=boolean
  maxp : simulink/Logic and Bit Operations/Compare To Constant  relop=<=  const=Estimator.pos.ofPitchRollMax  OutDataTypeStr=boolean
  maxp2 : simulink/Logic and Bit Operations/Compare To Constant  relop=<=  const=Estimator.pos.ofPQHovMax  OutDataTypeStr=boolean
  maxq : simulink/Logic and Bit Operations/Compare To Constant  relop=<=  const=Estimator.pos.ofPitchRollMax  OutDataTypeStr=boolean
  maxq2 : simulink/Logic and Bit Operations/Compare To Constant  relop=<=  const=Estimator.pos.ofPQHovMax  OutDataTypeStr=boolean
  maxw1 : simulink/Logic and Bit Operations/Compare To Constant  relop=<=  const=Estimator.pos.ofPQMax  OutDataTypeStr=boolean
  maxw2 : simulink/Logic and Bit Operations/Compare To Constant  relop=<=  const=Estimator.pos.ofPQMax  OutDataTypeStr=boolean
  maxw3 : simulink/Logic and Bit Operations/Compare To Constant  relop=<=  const=Estimator.pos.deltaDXYMax  OutDataTypeStr=boolean
  maxw4 : simulink/Logic and Bit Operations/Compare To Constant  relop=<=  const=Estimator.pos.deltaDXYMax  OutDataTypeStr=boolean
  minHeightforOF : simulink/Logic and Bit Operations/Compare To Constant  relop=<=  const=Estimator.pos.opticalFlowZMax  OutDataTypeStr=boolean
  enable_flag : Outport  VectorParamsAs1DForOutWhenUnconnected=off
  wires:
  minHeightforOF/1 -> Logical Operator3/4
  IIRgyroz/1 -> DiscreteDerivative/1
  Mux5/1 -> Demux1/1, Demux4/1, IIRgyroz/1
  maxw4/1 -> Logical Operator3/3
  maxw3/1 -> Logical Operator3/2
  dxyOF_datin/1 -> Add/1
  Demux3/2 -> Abs9/1
  Demux3/1 -> Abs8/1
  dxy_estimin/1 -> Add/2
  Add/1 -> Demux3/1
  Abs9/1 -> maxw4/1
  Abs8/1 -> maxw3/1
  Logical Operator2/1 -> Logical Operator3/1
  Logical Operator3/1 -> enable_flag/1
  DiscreteDerivative/1 -> Demux2/1  "dpq"
  Demux2/2 -> Abs7/1
  Demux2/1 -> Abs6/1
  Abs7/1 -> maxdw2/1
  Abs6/1 -> maxdw1/1
  Logical Operator1/1 -> Logical Operator2/2
  Demux1/2 -> Abs5/1
  Demux1/1 -> Abs4/1
  Abs5/1 -> maxq2/1
  Abs4/1 -> maxp2/1
  Abs3/1 -> maxq/1
  Abs2/1 -> maxp/1
  Demux4/2 -> Abs1/1
  Demux4/1 -> Abs/1
  Abs1/1 -> maxw2/1
  Abs/1 -> maxw1/1
  Z_estimin/1 -> minHeightforOF/1
  Logical Operator/1 -> Logical Operator2/1
  maxw1/1 -> Logical Operator/3
  Bus Selector/1 -> Mux5/1  "<p>"
  Selectpitchroll/1 -> Demux5/1
  sensorIMU_datin/1 -> Bus Selector/1
  maxq2/1 -> Logical Operator1/2
  Bus Selector/2 -> Mux5/2  "<q>"
  maxp/1 -> Logical Operator/1
  maxw2/1 -> Logical Operator/4
  orient_estimin/1 -> Selectpitchroll/1
  maxdw1/1 -> Logical Operator/5
  maxdw2/1 -> Logical Operator/6
  maxq/1 -> Logical Operator/2
  Demux5/1 -> Abs2/1
  Demux5/2 -> Abs3/1
  maxp2/1 -> Logical Operator1/1

== system flightControlSystem/Control System/State Estimator/XY Position Estimator/EstimatorVelocity/xy velocity w//o angular velocity compensation ==
  note: Optical flow raw readings are converted to velocity in m/s based on the estimated altitude
  optical_flow : Inport
  z_estimate : Inport  Port=2
  " " : Product  Inputs=**
  Compare To Constant : simulink/Logic and Bit Operations/Compare To Constant  relop=<  const=200*4  OutDataTypeStr=boolean
  Counter Free-Running : simulink/Sources/Counter Free-Running  NumBits=32  tsamp=-1
  Gain : Gain  Gain=-1
  Select dxy : Selector  InputPortWidth=3  IndexOptions=Index vector (dialog)  Indices=[1 2]  OutputSizes=1
  Switch : Switch  Criteria=u2 > Threshold
  opticalFlowErrorCorrect : Gain  Gain=1.15
  optical_flow_dx_dy : Outport
  wires:
  Select dxy/1 -> optical_flow_dx_dy/1  "optical_flow_dx_dy"
  " "/1 -> opticalFlowErrorCorrect/1
  opticalFlowErrorCorrect/1 -> Switch/3
  Gain/1 -> " "/2
  Switch/1 -> Select dxy/1
  Counter Free-Running/1 -> Compare To Constant/1
  Compare To Constant/1 -> Switch/2
  optical_flow/1 -> " "/1, Switch/1
  z_estimate/1 -> Gain/1

== matlab function flightControlSystem/Control System/Path Planning/Non linear Path Planner/parameter_setting ==
  data: circle_count input; CHANGE_DERIVATIVE_ERROR_THRESHOLD output; CHANGE_DERIVATIVE_ERROR_THRESHOLD_CURVE parameter; CHANGE_DERIVATIVE_ERROR_THRESHOLD_STRAIGHT parameter
function CHANGE_DERIVATIVE_ERROR_THRESHOLD = parametersetting(...
    circle_count,CHANGE_DERIVATIVE_ERROR_THRESHOLD_CURVE,...
CHANGE_DERIVATIVE_ERROR_THRESHOLD_STRAIGHT)

if circle_count <=1
   CHANGE_DERIVATIVE_ERROR_THRESHOLD = CHANGE_DERIVATIVE_ERROR_THRESHOLD_STRAIGHT;
else
   CHANGE_DERIVATIVE_ERROR_THRESHOLD = CHANGE_DERIVATIVE_ERROR_THRESHOLD_CURVE;
end
end

== stateflow chart flightControlSystem/Control System/Path Planning/Non linear Path Planner/X_PLANNER/Chart1 ==
  state STATE [group]
    - TRACKING: The drone is tracking the lane or the end-marker.
    - LANDING: The drone is landing if the end-marker is detected and the error between the drone CoG and the middle
    point of the end-marker is less than MAX_ERROR_LANDING.
    - TRACK_DETECTED: The Image Processing System detected the lane.
    - END_MARKER_DETECTED: The Image Processing System detected the end-marker.
  state INPUT [group]
    - flag_track: flag raised when the track is detected by the Image Processing System.
    - flag_end_marker_to_controller: flag raised when the drone has to land.
    - lin_part: linear part of the path planner.
    - dev_part: derivative part of the path planner.
    - x_estimated: postion x estimated from the sensors.
    - flag_end_marker: flag raised when the land-marker is detected by the Image Processing System.
  state OUTPUT [group]
    - x_planned: x coordinate of the goal position.
  state LANDING
    during:
    x_planned=x_planned_stored;
  state END_MARKER_DETECTED
    entry:
    circle_count = circle_count + 1;
    during:
    x_planned = x_estimated + lin_part ;
    x_planned_stored = x_planned;
  state TAKE_OFF
    x_planned = 0;
  state LINE_DETECTED
    during:
    x_planned = x_estimated + lin_part + dev_part;
    x_planned_stored = x_planned;
  state LEAVE_MARKER
    during:
    x_planned = x_estimated +0.045 ;
  (default) -> TAKE_OFF : {circle_count = 0}
  END_MARKER_DETECTED -> LANDING : [flag_end_marker_to_controller==1]
  TAKE_OFF -> END_MARKER_DETECTED : [after(3,sec) && flag_end_marker == 1 ]
  LINE_DETECTED -> END_MARKER_DETECTED : [flag_end_marker == 1]
  LANDING -> LEAVE_MARKER : [after(5,sec) && flag_hover == 1 && circle_count <=2]
  LEAVE_MARKER -> LINE_DETECTED : [ flag_end_marker ==0&&flag_track ==1]
  data: dev_part input double; lin_part input double; x_planned output double; flag_end_marker_to_controller input double; x_estimated input double; flag_track input double; x_planned_stored local double; flag_end_marker input double; circle_count local double; flag_hover input

== matlab function flightControlSystem/Control System/Path Planning/Take off checker ==
  data: z_est input; flag_hover output; Z_LOW parameter; Z_HIGH parameter; FLAG_WAIT_FOR_HOVERING parameter
function flag_hover = height_checker(z_est, Z_LOW, Z_HIGH, FLAG_WAIT_FOR_HOVERING)
% This MATLAB function raise a flag when the drone is hovering by using the
% z_low and z_high variable which are threshold level expressed in meters. The output is a
% flag that permits the path planner to be activated and perform the
% trajectory tracking.
%
% Inputs:
% - z_low: low threshold height, in meters
% - z_high: high threshold height, in meters
% - z_est: estimation of drone's height 
% - FLAG_WAIT_FOR_HOVERING: the flag is used to decide if path planner is
% activie before or after drone takes off (TRUE/FALSE)
%
% Output:
% - flag_hover: the flag indicates the drone takes off successfully 
%and is ready for next state.

if FLAG_WAIT_FOR_HOVERING == 0
    
    if z_est < Z_LOW && z_est > Z_HIGH
        
        flag_hover = 1 ;
    else
        
        flag_hover = 0 ;
        
    end
    
else
    
    flag_hover = 1 ;
    
end

end

== matlab function flightControlSystem/Control System/Path Planning/MATLAB Function ==
  data: x_err_tr_s input; x_error output; y_err_tr_s input; x_err_ea input; y_err_ea input; flag_ea input; flag_ho input; y_error output; flag_tr_s input; x_err_tr_c input; y_err_tr_c input; flag_tr_c input; circle_count input; track_flag output
function [x_error, y_error,track_flag] = decision_making(x_err_tr_s, y_err_tr_s, x_err_ea, ...
    y_err_ea, flag_ea, flag_ho, flag_tr_s, x_err_tr_c, y_err_tr_c, flag_tr_c, circle_count)
% The MALTAB function sends the error along x- and y-axis to the drone 
% trajectory controller. When the "flag_ea" is low, the position errors
% are computed as the difference between the end-marker and the drone
% CoG. Instead, when the flag is high, the errors are computed by the
% Image Processing System.
%
% Inputs:
% - x_err_tr: tracking error along the x-axis. The error is expressed in 
% pixels.
% - y_err_tr: tracking error along the y-axis. The error is expressed in 
% pixels.
% - x_err_ea: position error along the x-axis when the end-marker is 
% detected. The error is expressed in pixels.
% - y_err_ea: position error along the y-axis when the end-marker is
% detected. The error is expressed in pixels.
% - flag_ea: the flag allows to check if the end-maker is recognized.
% - flag_ho: the flag allows to check if the drone is able to fly.
%   
% Outputs
% - x_error: error between the drone CoG and the track/end-marker along the 
% x-axis. The error is expressed in pixels.
% - y_error: error between the drone CoG and the track/end-marker along the
% y-axis. The error is expressed in pixels

if flag_ho == 1
    
    if flag_ea == 1
        
        x_error=x_err_ea;
        y_error=y_err_ea;
        track_flag = 0;
             
    elseif circle_count <= 1
        
        x_error=x_err_tr_s;
        y_error=y_err_tr_s;
        track_flag = flag_tr_s;
    else
        x_error=x_err_tr_c;
        y_error=y_err_tr_c;
        track_flag = flag_tr_c;
        
    end
    
else
    
    x_error=0;
    y_error=0;
    track_flag = 0;
    
end
    
end

== matlab function flightControlSystem/Image Processing System/Waypoints_straight ==
  data: frame input; error_y_track output; x_ref_prev input; y_ref_prev input; flag_track_prev input; error_x_track output; orientation_track output; flag_track output boolean; MIN_RADIUS_CROWN_STRAIGHT parameter; MAX_RADIUS_CROWN_STRAIGHT parameter; FOV_STRAIGHT parameter; COG_X parameter; COG_Y parameter
function [error_y_track, error_x_track, orientation_track, flag_track] = ...
error_pixel_generator(frame, x_ref_prev, y_ref_prev, flag_track_prev, ...
MIN_RADIUS_CROWN_STRAIGHT, MAX_RADIUS_CROWN_STRAIGHT, FOV_STRAIGHT, COG_X, COG_Y)
% The MATLAB function computes the error along x and y-axis between
% the drone COG (Center of Gravity) and the point of the track extract 
% by using of a crown circular mask. This errors is later used by the Path 
% Planner for the lane tracking  
%
%
% Inputs:
% - frame: binarized frame
% - x_ref_prev: previous value of the tracking point along the x-axis of 
% the track line. It is used as a reference for tracking the path.
% - y_ref_prev: previous value of the tracking point along the y-axis of 
% the track line. It is used as a reference for tracking the path.                                                                                                                                              
% - flag_track_prev: previous value assumed by the flag variablle, i.e., 
% the previous state of the drone (over the track / not over the track).
%
%
% Outputs:
% - error_y_track: error between the CoG of the drone and a point of the 
% lane in the forward direction along the y-axis. It is expressed in
% pixels.
% - error_x_track: error between the CoG of the drone and a point of the 
% lane in the forward direction along the x-axis. It is expressed in pixels. 
% - flag_track: it indicates if the drone is currently over the track (TRUE).
% - yaw: the heading angle of the track in the image plane.
%
%
% Parameters:
% - MIN_RADIUS_CROWN: minimum value of the radius of the crown mask. It is
% expressed in pixels.
% - MAX_RADIUS_CROWN: maximum value of the radius of the crown mask. It is
% expressed in pixels.
% - FOV: a portion of the crown used to detect the lane. It is expressed in
% radians.
% - COG_X: position of the drone CoG along x-axis of the reference frame.
% - COG_Y: position of the drone CoG along y-axis of the reference frame.

persistent x_accumulator
persistent y_accumulator
persistent pixel_count

if isempty(x_accumulator)
    x_accumulator = 0;
end

if isempty(y_accumulator)
    y_accumulator = 0;
end

if isempty(pixel_count)
    pixel_count = 0;
end

% the previous value of the heading angle of the lane 
orientation_track = atan2(-x_ref_prev,y_ref_prev); 
orientation_track = mod(orientation_track,2*pi);

% checking if the drone is over the lane
if flag_track_prev     

    % the set of pixels inside the crown mask
    for i = (COG_X-MAX_RADIUS_CROWN_STRAIGHT):(COG_X+MAX_RADIUS_CROWN_STRAIGHT) 

        for j = (COG_Y-MAX_RADIUS_CROWN_STRAIGHT):(COG_Y+MAX_RADIUS_CROWN_STRAIGHT)

            norm = sqrt(((i-(COG_X-0.5))^2)+((j-(COG_Y-0.5))^2));

            if norm >= MIN_RADIUS_CROWN_STRAIGHT && norm <= MAX_RADIUS_CROWN_STRAIGHT 

                axis_x = (i-(COG_X-0.5));
                axis_y = (j-(COG_Y-0.5));
                yaw_point_temp = atan2(axis_x,axis_y);


                yaw_point_temp_2 = mod(yaw_point_temp,2*pi);

                % a portion of the crown mask depending on the FOV
                threshold_1 = mod((orientation_track+(pi/FOV_STRAIGHT)),2*pi);

                threshold_2 = mod((orientation_track-(pi/FOV_STRAIGHT)),2*pi);

                if threshold_1 < threshold_2

                    flag_threshold = ...
                        (yaw_point_temp_2 <= 2*pi  && yaw_point_temp_2 >= threshold_2) ...
                        || (yaw_point_temp_2 <= threshold_1  && yaw_point_temp_2 >= 0);

                else

                    flag_threshold = ...
                        yaw_point_temp_2 <= threshold_1  && yaw_point_temp_2 >= threshold_2;

                end

                if flag_threshold
 
                    if frame(i,j)==1 
                        
                        pixel_count = pixel_count + 1;
                        x_accumulator = x_accumulator + i;
                        y_accumulator = y_accumulator + j;

                    end

                end

            end

        end
    end
    
else
    % checking for the initial heading angle of the lane. It can be 
    % different from the heading angle of the drone
    for i = (COG_X-MAX_RADIUS_CROWN_STRAIGHT):(COG_X+MAX_RADIUS_CROWN_STRAIGHT)

        for j = (COG_Y-MAX_RADIUS_CROWN_STRAIGHT):(COG_Y+MAX_RADIUS_CROWN_STRAIGHT)
            
            norm=sqrt(((i-(COG_X-0.5))^2)+((j-(COG_Y-0.5))^2));

            if norm>=MIN_RADIUS_CROWN_STRAIGHT && norm <= MAX_RADIUS_CROWN_STRAIGHT 

                 axis_x = (i-(COG_X-0.5));
                 axis_y = (j-(COG_Y-0.5));
                if frame(i,j)==1 
                    pixel_count=pixel_count +1;
                    x_accumulator=x_accumulator+i;
                    y_accumulator=y_accumulator+j;
                end
            end
        end
    end
end

% calculating the medium point of the lane as output of the mask
x_ref_temp = -(round(x_accumulator/pixel_count)-COG_X);
y_ref_temp = (round(y_accumulator/pixel_count)-COG_Y);

% when there is no track, the x_ref_temp and y_ref_temp variables are NaN.
% Below is the code for fix the issue.

if isnan(x_ref_temp)
    
    % if the computer vision algorithm does not detect the track, the 
    % drone position does not change
    error_x_track = 0 ;
    flag_error_x = false;
    
else
    
    % if the computer vision algorithm detects the track, a new position 
    % is computed for the tracking problem
    flag_error_x = true;
    error_x_track = x_ref_temp;
    
end

% As for the x coordinate
if isnan(y_ref_temp)
    
    error_y_track = 0 ;
    flag_error_y = false;
    
else
    
    error_y_track = y_ref_temp;
    flag_error_y=true ;
    
end

% checking if the drone is over the lane
flag_track = flag_error_x || flag_error_y;

% reset of the persistent variables
pixel_count = 0;
x_accumulator = 0;
y_accumulator = 0;

end
